simulink model "Heatpumptest"  (R2022a)
settings: Solver=ode1be  StartTime=0.0  StopTime=10.0  FixedStep=0.05  RelTol=1e-3
libraries: kif2 x4, simulink x3
settings Model: Creator=Felhasználó  LastModifiedBy=Felhasználó

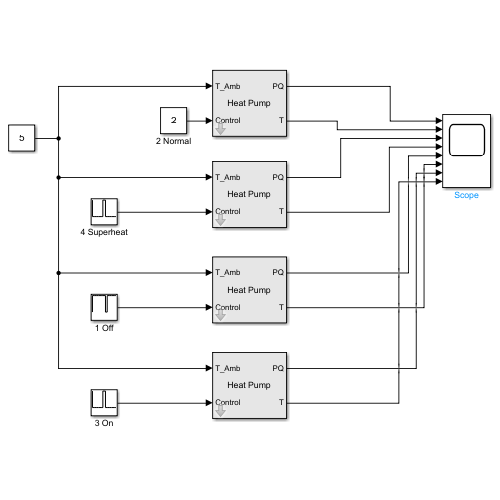
[thumbnail: Simulink's stored preview of the top-level diagram]
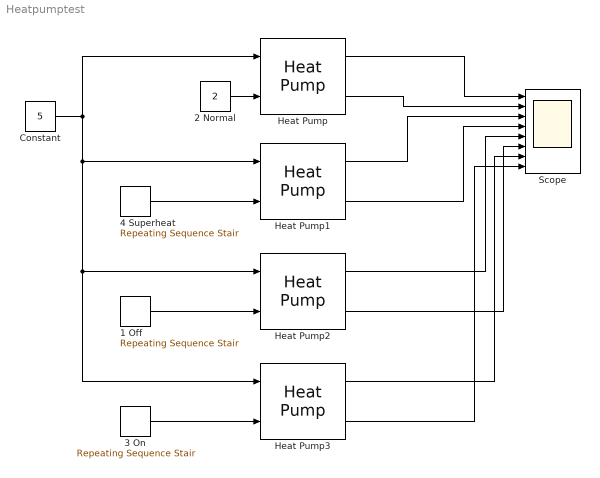
== system Heatpumptest ==
  1 Off : simulink/Sources/Repeating Sequence Stair  OutValues=[2 2 2 2 2 2 1 2 2 2 2].'  tsamp=1  OutMin=[]  OutMax=[]  OutDataTypeStr=double  OutputDataTypeScalingMode=double  OutDataType=fixdt(0,8)  ConRadixGroup=Best Precision: Vector-wise  OutScaling=2^-12
  2 Normal : Constant  Value=2
  3 On : simulink/Sources/Repeating Sequence Stair  OutValues=[2 2 2 2 2 3 2 2 2 2 2].'  tsamp=1  OutMin=[]  OutMax=[]  OutDataTypeStr=double  OutputDataTypeScalingMode=double  OutDataType=fixdt(0,8)  ConRadixGroup=Best Precision: Vector-wise  OutScaling=2^-12
  4 Superheat : simulink/Sources/Repeating Sequence Stair  OutValues=[2 2 2 2 2 4 2 2 2 2 2].'  tsamp=1  OutMin=[]  OutMax=[]  OutDataTypeStr=double  OutputDataTypeScalingMode=double  OutDataType=fixdt(0,8)  ConRadixGroup=Best Precision: Vector-wise  OutScaling=2^-12
  Constant : Constant  Value=5
  Heat Pump{,1..3} (4 alike) : kif2/Heat Pump  MFSystemSampleTime=0.05  tequiv=3  P_HP=3800  Tset=21  T_init=21  C=5940  H=192  ASHP=on  Mode=on  coeffs=[0.0012, -0.18, 8.6712]  cosfi=0.9
      settings: SourceProductName=KIF2 Library
  Scope : Scope  NumInputPorts=8
  wires:
  Constant/1 -> Heat Pump/1, Heat Pump2/1, Heat Pump3/1, Heat Pump1/1
  2 Normal/1 -> Heat Pump/2
  4 Superheat/1 -> Heat Pump1/2
  Heat Pump/1 -> Scope/1
  Heat Pump1/1 -> Scope/3
  Heat Pump/2 -> Scope/2
  Heat Pump1/2 -> Scope/4
  1 Off/1 -> Heat Pump2/2
  Heat Pump2/2 -> Scope/6
  Heat Pump2/1 -> Scope/5
  Heat Pump3/1 -> Scope/7
  Heat Pump3/2 -> Scope/8
  3 On/1 -> Heat Pump3/2
